simulink model "DataAnalysis_v2"  (Simulink 7.6)
settings: Solver=FixedStepDiscrete  StartTime=0.0  StopTime=0  RelTol=1e-3
undefined symbols (not defined in the file or in its folder): gray, Rec, SDTV
libraries: vipconversions x1, vipsnks x1, vipsrcs x1, viptextngfix x1
settings Model: Creator=Thing 1  LastModifiedBy=auvt
settings RTWCC: TargetLang=C++

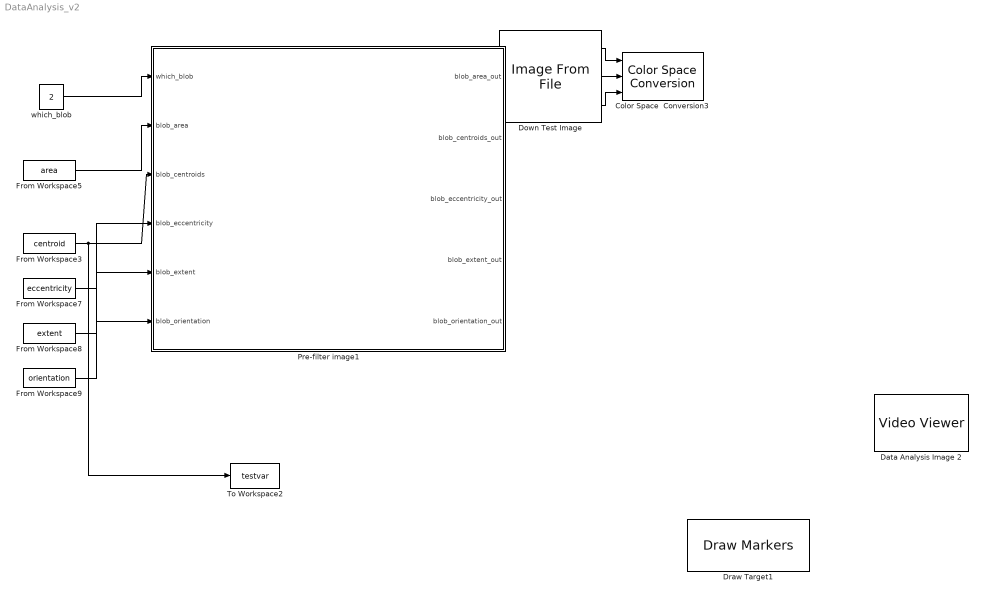
== system DataAnalysis_v2 ==
  Color Space  Conversion3 : vipconversions/Color Space  Conversion  conversion=Obsolete  conversionActive=R'G'B' to HSV  wp_str=D65  rec=Rec. 601 (SDTV)  sys=1125/60/2:1  imagePorts=Separate color signals
  Data Analysis Image 2 : vipsnks/Video Viewer  DialogControllerArgs=DataTag1  inputType=Obsolete7b  imagePorts=One multidimensional signal  useColorMap=off  colormapValue=gray(256)  specRange=off  minInputVal=0  maxInputVal=255  FigPos=[1622 595 492 307]  AxisZoom=on  trueSizedOnce=off  OpenAtMdlStart=on
  Down Test Image : vipsrcs/Image From File  Tag=vipblks_nd  DialogController=vipDDGCreate  DialogControllerArgs=DataTag2  SystemSampleTime=-1  FileName=/home/auvt/auvc/src/vision/Test_Images/path9.bmp  imagePorts=Separate color signals  Ts=-1  ImageDataType=double  Signed=on  WordLength=16  sdImageDataType=uint(8)  FractionLengthMode=User-defined  FractionLength=15  OutPortLabels=R|G|B
  Draw Target1 : viptextngfix/Draw Markers  DialogController=vipDDGCreate  DialogControllerArgs=DataTag3  shape=X-mark  size=7  fill=off  fillClrSource=Specify via dialog  display=White  intensity=200  color=[0 0 0]  opacity=0.6  viewport=Entire image  antialiasing=off  inType=Obsolete  imagePorts=One multidimensional signal  prodOutputMode=Binary point scaling  prodOutputWordLength=32  prodOutputFracLength=14  memoryMode=Specify word length  memoryWordLength=16  memoryFracLength=15  roundingMode=Floor  overflowMode=off
  From Workspace3 : FromWorkspace  VariableName=centroid  SampleTime=0
  From Workspace5 : FromWorkspace  VariableName=area  SampleTime=0
  From Workspace7 : FromWorkspace  VariableName=eccentricity  SampleTime=0
  From Workspace8 : FromWorkspace  VariableName=extent  SampleTime=0
  From Workspace9 : FromWorkspace  VariableName=orientation  SampleTime=0
  Pre-filter image1 : Stateflow chart  TreatAsAtomicUnit=on
  To Workspace2 : ToWorkspace  VariableName=testvar  SampleTime=-1  SaveFormat=Array
  which_blob : Constant  Value=2  SampleTime=-1
  wires:
  which_blob/1 -> Pre-filter image1/1(which_blob)
  From Workspace3/1 -> Pre-filter image1/3(blob_centroids), To Workspace2/1
  From Workspace5/1 -> Pre-filter image1/2(blob_area)
  From Workspace7/1 -> Pre-filter image1/4(blob_eccentricity)
  From Workspace8/1 -> Pre-filter image1/5(blob_extent)
  From Workspace9/1 -> Pre-filter image1/6(blob_orientation)
  ? -> Data Analysis Image 2/1
  Down Test Image/1 -> Color Space  Conversion3/1
  Down Test Image/2 -> Color Space  Conversion3/2
  Down Test Image/3 -> Color Space  Conversion3/3

== matlab function Pre-filter image1 ==
  data: which_blob input double; blob_area input double; blob_centroids input double; blob_eccentricity input double; blob_extent input double; blob_orientation input double; blob_area_out output double; blob_centroids_out output double; blob_eccentricity_out output double; blob_extent_out output double; blob_orientation_out output double
function [blob_area_out, blob_centroids_out, blob_eccentricity_out, blob_extent_out, blob_orientation_out] = chooseBlob(which_blob, blob_area, blob_centroids, blob_eccentricity, blob_extent, blob_orientation)
%#eml

blob_area_out = blob_area(which_blob);
blob_centroids_out = blob_centroids(:,:);
blob_eccentricity_out = blob_eccentricity(which_blob,:);
blob_extent_out = blob_extent(which_blob,:);
blob_orientation_out = blob_orientation(which_blob,:);




return
